simulink model "playground"  (R2024a)
settings: Solver=ode45  StartTime=0.0  StopTime=10.0  FixedStep=0.001  RelTol=1e-3
values from neighbouring files (symbols this model uses):
  a_r = 1.14 * 10^(-7)    (= 1.14e-07)    [start.m]    (also in startEnglPaper.m = 0.033; startReduced.m)
  a_rS = b    (= 0.033)    [startEnglPaper.m]
  A_x = 0.25    [playgrounMat.m]    (also in start.m; startEnglPaper.m; startReduced.m)
  A_y = 0.25    [playgrounMat.m]    (also in start.m; startEnglPaper.m; startReduced.m)
  A_z = 0.25    [playgrounMat.m]    (also in start.m; startEnglPaper.m; startReduced.m)
  b = 1.14 * 10^(-7)    (= 1.14e-07)    [start.m]    (also in startEnglPaper.m = 0.033; startReduced.m)
  g = 9.81    [playgrounMat.m]    (also in start.m; startEnglPaper.m; startReduced.m)
  gamma_d = pi/3    (= 1.0471975512)    [start.m]    (also in startReduced.m)
  I_r = 5.38 * 10 ^ (-5)    (= 5.38e-05)    [start.m]    (also in startEnglPaper.m = 3.38e-05; startReduced.m)
  I_x = 0.0151    [start.m]    (also in startEnglPaper.m = 0.004856; startReduced.m)
  I_y = 0.253    [start.m]    (also in startEnglPaper.m = 0.004856; startReduced.m)
  I_z = 0.0151    [start.m]    (also in startEnglPaper.m = 0.008801; startReduced.m)
  IrS = 5.38 * 10^(-5)    (= 5.38e-05)    [startEnglPaper.m]
  IxS = 0.0151    [startEnglPaper.m]
  IyS = IxS    (= 0.0151)    [startEnglPaper.m]
  IzS = 0.0253    [startEnglPaper.m]
  k = 1.045 * 10^(-11)    (= 1.045e-11)    [start.m]    (also in startEnglPaper.m = 2.98e-06; startReduced.m)
  K_gamma_D1 = K(1)    [playgrounMat.m]
  K_gamma_I1 = K(3)    [playgrounMat.m]
  K_gamma_P1 = K(2)    [playgrounMat.m]
  K_phi_D1 = 0.047    [startEnglPaper.m]
  K_phi_D11 = 0.093    [startEnglPaper.m]
  K_phi_D2 = 9.6    [startEnglPaper.m]
  K_phi_D22 = 19.2    [startEnglPaper.m]
  K_phi_DS = 0.14    [startEnglPaper.m]
  K_phi_I11 = 1.27    [startEnglPaper.m]
  K_phi_I22 = 262.144    [startEnglPaper.m]
  K_phi_P1 = 0.11    [startEnglPaper.m]
  K_phi_P11 = 0.5966    [startEnglPaper.m]
  K_phi_P2 = 23.04    [startEnglPaper.m]
  K_phi_P22 = 122.88    [startEnglPaper.m]
  K_phi_PS = 0.35    [startEnglPaper.m]
  K_psi_D = 40    [start.m]    (also in startEnglPaper.m = 9.6; startReduced.m)
  K_psi_D1 = 0.0844    [startEnglPaper.m]
  K_psi_D2 = 9.6    [startEnglPaper.m]
  K_psi_D22 = 19.2    [startEnglPaper.m]
  K_psi_DS = 0.24    [startEnglPaper.m]
  K_psi_I22 = 262.144    [startEnglPaper.m]
  K_psi_P = 143    [start.m]    (also in startEnglPaper.m = 23.04; startReduced.m)
  K_psi_P1 = 0.202    [startEnglPaper.m]
  K_psi_P2 = 23.04    [startEnglPaper.m]
  K_psi_P22 = 122.88    [startEnglPaper.m]
  K_psi_PS = 0.58    [startEnglPaper.m]
  K_theta_D = 58    [start.m]    (also in startEnglPaper.m = 9.6; startReduced.m)
  K_theta_D1 = 0.047    [startEnglPaper.m]
  K_theta_D2 = 9.6    [startEnglPaper.m]
  K_theta_D22 = 19.2    [startEnglPaper.m]
  K_theta_DS = 0.14    [startEnglPaper.m]
  K_theta_I22 = 262.144    [startEnglPaper.m]
  K_theta_P = 141    [start.m]    (also in startEnglPaper.m = 23.04; startReduced.m)
  K_theta_P1 = 0.11    [startEnglPaper.m]
  K_theta_P2 = 23.04    [startEnglPaper.m]
  K_theta_P22 = 122.88    [startEnglPaper.m]
  K_theta_PS = 0.35    [startEnglPaper.m]
  K_y_D = 13.58    [start.m]    (also in startReduced.m)
  K_y_P = 33.18    [start.m]    (also in startReduced.m)
  K_z_D1 = 4.42    [startEnglPaper.m]
  K_z_D2 = 4.42/m + A_z/m    (= 9.60905349794)    [startEnglPaper.m]
  K_z_DS = 13.58    [startEnglPaper.m]
  K_z_P1 = 11.2    [startEnglPaper.m]
  K_z_P2 = 11.2/m + A_z/m    (= 23.5596707819)    [startEnglPaper.m]
  K_z_PS = 33.18    [startEnglPaper.m]
  kl = 3 * 10^(-6)    (= 3e-06)    [startEnglPaper.m]
  l = 0.225    [start.m]    (also in startEnglPaper.m; startReduced.m)
  m = 1.44    [playgrounMat.m]    (also in start.m; startEnglPaper.m = 0.486; startReduced.m)
  m_s = [1/4 0 -1/(2*l) -1/(4*a_r); 1/4 -1/(2*l) 0 1/(4*a_r); 1/4 0 1/(2*l) -1/(4*a_r); 1/4 1/(2*l) 0 1/(4*a_r)]    [start.m]    (also in startReduced.m)
  mS = 1.44    [startEnglPaper.m]
  phi_d = 0.2    [startEnglPaper.m]
  phi_DesS = 0.2    [startEnglPaper.m]
  phi_init = 0    [startEnglPaper.m]
  phi_iS = 0;   deg2rad(10)    [startEnglPaper.m]
  psi_d = pi/5    (= 0.628318530718)    [start.m]    (also in startEnglPaper.m = 0.15; startReduced.m)
  psi_DesS = 0.15    [startEnglPaper.m]
  psi_init = 0    [startEnglPaper.m]
  psi_iS = 0    [startEnglPaper.m]
  theta_d = pi/4    (= 0.785398163397)    [start.m]    (also in startEnglPaper.m = 0.3; startReduced.m)
  theta_DesS = -0.1 * -3    (= 0.3)    [startEnglPaper.m]
  theta_init = 0    [startEnglPaper.m]
  theta_iS = 0    [startEnglPaper.m]
  x_init = 0    [startEnglPaper.m]
  x_iS = 0    [startEnglPaper.m]
  y_init = 0    [startEnglPaper.m]
  y_iS = 0    [startEnglPaper.m]
  z_d = 0.05 * 0    (= 0)    [startEnglPaper.m]
  z_DesS = 0.1    [startEnglPaper.m]
  z_init = 0    [startEnglPaper.m]
  z_iS = 0.0    (= 0)    [startEnglPaper.m]
undefined symbols (not defined in the file or in its folder): m_s_my
libraries: slpidlib x14
(part 3 of 4)

== system playground/CHANGE_PID/CONTROLLER/PD regulator theta ==
  theta : Inport
  (theta)' : Inport  Port=2
  Altitude controller : slpidlib/PID Controller  Controller=PID  Form=Parallel  TimeDomain=Continuous-time  UseExternalTs=off  SampleTime=-1  IntegratorMethod=Forward Euler  FilterMethod=Forward Euler  ControllerParametersSource=internal  P=K_theta_P1  I=0  UseKiTs=off  D=K_theta_D1  UseExternalDerivativeSource=off  N=100  UseFilter=on  TunerSelectOption=Transfer Function Based (PID Tuner App)  InitialConditionSource=internal  InitialConditionForIntegrator=0  InitialConditionForFilter=0  DifferentiatorICPrevScaledInput=0  ExternalReset=none  TrackingMode=off  Kt=1  LimitOutput=on  SatLimitsSource=internal  UpperSaturationLimit=5  LowerSaturationLimit=-5  LinearizeAsGain=on  AntiWindupMode=none  Kb=1  LimitIntegrator=off  UpperIntegratorSaturationLimit=inf  LowerIntegratorSaturationLimit=-inf  POutMin=[]  POutMax=[]  IOutMin=[]  IOutMax=[]  DOutMin=[]  DOutMax=[]  NOutMin=[]  NOutMax=[]  SumOutMin=[]  SumOutMax=[]  SaturationOutMin=[]  SaturationOutMax=[]  PParamMin=[]  PParamMax=[]  IParamMin=[]  IParamMax=[]  DParamMin=[]  DParamMax=[]  NParamMin=[]  NParamMax=[]  KbParamMin=[]  KbParamMax=[]  KtParamMin=[]  KtParamMax=[]  KbOutMin=[]  KbOutMax=[]  KtOutMin=[]  KtOutMax=[]  IntegratorOutMin=[]  IntegratorOutMax=[]  FilterOutMin=[]  FilterOutMax=[]  SumI1OutMin=[]  SumI1OutMax=[]  SumI2OutMin=[]  SumI2OutMax=[]  SumI3OutMin=[]  SumI3OutMax=[]  SumI4OutMin=[]  SumI4OutMax=[]  SumDOutMin=[]  SumDOutMax=[]  DifferentiatorOutMin=[]  DifferentiatorOutMax=[]  FilterDiffOutCoefMin=[]  FilterDiffOutCoefMax=[]  ReciprocalOutMin=[]  ReciprocalOutMax=[]  SumDenOutMin=[]  SumDenOutMax=[]  SumNumOutMin=[]  SumNumOutMax=[]  DivideOutMin=[]  DivideOutMax=[]  UdiffTsProdOutMin=[]  UdiffTsProdOutMax=[]  NTsProdOutMin=[]  NTsProdOutMax=[]  UintegralTsProdOutMin=[]  UintegralTsProdOutMax=[]  UngainTsProdOutMin=[]  UngainTsProdOutMax=[]  ClampingZeroOutDataTypeStr=Inherit: Inherit via back propagation  ClampingZeroOutMin=[]  ClampingZeroOutMax=[]  FilterDenConstantOutDataTypeStr=Inherit: Inherit via back propagation  FilterDenConstantOutMin=[]  FilterDenConstantOutMax=[]  PCopyOutDataTypeStr=Inherit: Inherit via back propagation  PCopyOutMin=[]  PCopyOutMax=[]  NCopyOutDataTypeStr=Inherit: Inherit via back propagation  NCopyOutMin=[]  NCopyOutMax=[]  IntegratorContinuousStateAttributes=''  IntegratorStateMustResolveToSignalObject=off  IntegratorRTWStateStorageClass=Auto  FilterContinuousStateAttributes=''  FilterStateMustResolveToSignalObject=off  FilterRTWStateStorageClass=Auto  ParallelPVariant=InternalParameters  IdealPVariant=Disabled  IVariant=InternalParameters  DVariant=InternalParameters  IntegratorVariant=Continuous  SatVariant=Enabled  AWVariant=Passthrough  PCopyVariant=Disabled  TRVariant=Disabled  FdbkBlocksVariant=Forward  IdealPFdbkVariant=Disabled  SatFdbkVariant=Disabled  DerivativeFilterVariant=ContFilter  NVariant=InternalParameters  NCopyVariant=Disabled  FilterICVariant=InternalICsFilter  IntegratorICVariant=InternalICs  ExternalResetVariant=Disabled  TRSumVariant=Passthrough  SumFdbkVariant=Disabled  SumVariant=Sum_PID  TsampFilterVariant=InternalTs  TsampNgainVariant=Passthrough  TsampIntegralVariant=Disabled_SignalSpec  ExternalSaturationOutDataTypeStr=Inherit: Same as second input  DerivativeSourceVariant=ErrorSignal
  Constant : Constant  Value=I_y/I_y
  Constant1 : Constant  Value=K_theta_D1
  Constant2 : Constant  Value=theta_d
  Constant4 : Constant  Value=K_theta_P1
  Constant5 : Constant  Value=theta_d
  Current x{,1..3} (4 alike) : Display
  Derivative : Derivative
  Product : Product
  Product1 : Product
  Product2 : Product
  Sum : Sum  Inputs=++|
  Sum1 : Sum  Inputs=|+-
  Sum2 : Sum  Inputs=|+-
  tau_theta : Outport
  wires:
  Product/1 -> Current x3/1, Sum/1
  Constant1/1 -> Product/1
  Product1/1 -> Current x2/1, Sum/2
  Sum1/1 -> Product/2
  Constant4/1 -> Product1/1
  theta/1 -> Sum2/2
  Constant5/1 -> Sum2/1
  Derivative/1 -> Sum1/1
  Constant2/1 -> Derivative/1
  (theta)'/1 -> Sum1/2
  Sum2/1 -> Current x/1, Altitude controller/1, Product1/2
  Product2/1 -> tau_theta/1  "tau_theta"
  Constant/1 -> Product2/2
  Altitude controller/1 -> Current x1/1, Product2/1

== system playground/ST_constants_no_IX/CONTROLLER/PD regulator draft ==
  phi : Inport
  theta : Inport  Port=2
  z : Inport  Port=3
  Altitude controller : slpidlib/PID Controller  Controller=PID  Form=Parallel  TimeDomain=Continuous-time  UseExternalTs=off  SampleTime=-1  IntegratorMethod=Forward Euler  FilterMethod=Forward Euler  ControllerParametersSource=internal  P=K_z_PS  I=0  UseKiTs=off  D=K_z_DS  UseExternalDerivativeSource=off  N=100  UseFilter=on  TunerSelectOption=Transfer Function Based (PID Tuner App)  InitialConditionSource=internal  InitialConditionForIntegrator=0  InitialConditionForFilter=0  DifferentiatorICPrevScaledInput=0  ExternalReset=none  TrackingMode=off  Kt=1  LimitOutput=on  SatLimitsSource=internal  UpperSaturationLimit=5  LowerSaturationLimit=-5  LinearizeAsGain=on  AntiWindupMode=none  Kb=1  LimitIntegrator=off  UpperIntegratorSaturationLimit=inf  LowerIntegratorSaturationLimit=-inf  POutMin=[]  POutMax=[]  IOutMin=[]  IOutMax=[]  DOutMin=[]  DOutMax=[]  NOutMin=[]  NOutMax=[]  SumOutMin=[]  SumOutMax=[]  SaturationOutMin=[]  SaturationOutMax=[]  PParamMin=[]  PParamMax=[]  IParamMin=[]  IParamMax=[]  DParamMin=[]  DParamMax=[]  NParamMin=[]  NParamMax=[]  KbParamMin=[]  KbParamMax=[]  KtParamMin=[]  KtParamMax=[]  KbOutMin=[]  KbOutMax=[]  KtOutMin=[]  KtOutMax=[]  IntegratorOutMin=[]  IntegratorOutMax=[]  FilterOutMin=[]  FilterOutMax=[]  SumI1OutMin=[]  SumI1OutMax=[]  SumI2OutMin=[]  SumI2OutMax=[]  SumI3OutMin=[]  SumI3OutMax=[]  SumI4OutMin=[]  SumI4OutMax=[]  SumDOutMin=[]  SumDOutMax=[]  DifferentiatorOutMin=[]  DifferentiatorOutMax=[]  FilterDiffOutCoefMin=[]  FilterDiffOutCoefMax=[]  ReciprocalOutMin=[]  ReciprocalOutMax=[]  SumDenOutMin=[]  SumDenOutMax=[]  SumNumOutMin=[]  SumNumOutMax=[]  DivideOutMin=[]  DivideOutMax=[]  UdiffTsProdOutMin=[]  UdiffTsProdOutMax=[]  NTsProdOutMin=[]  NTsProdOutMax=[]  UintegralTsProdOutMin=[]  UintegralTsProdOutMax=[]  UngainTsProdOutMin=[]  UngainTsProdOutMax=[]  ClampingZeroOutDataTypeStr=Inherit: Inherit via back propagation  ClampingZeroOutMin=[]  ClampingZeroOutMax=[]  FilterDenConstantOutDataTypeStr=Inherit: Inherit via back propagation  FilterDenConstantOutMin=[]  FilterDenConstantOutMax=[]  PCopyOutDataTypeStr=Inherit: Inherit via back propagation  PCopyOutMin=[]  PCopyOutMax=[]  NCopyOutDataTypeStr=Inherit: Inherit via back propagation  NCopyOutMin=[]  NCopyOutMax=[]  IntegratorContinuousStateAttributes=''  IntegratorStateMustResolveToSignalObject=off  IntegratorRTWStateStorageClass=Auto  FilterContinuousStateAttributes=''  FilterStateMustResolveToSignalObject=off  FilterRTWStateStorageClass=Auto  ParallelPVariant=InternalParameters  IdealPVariant=Disabled  IVariant=InternalParameters  DVariant=InternalParameters  IntegratorVariant=Continuous  SatVariant=Enabled  AWVariant=Passthrough  PCopyVariant=Disabled  TRVariant=Disabled  FdbkBlocksVariant=Forward  IdealPFdbkVariant=Disabled  SatFdbkVariant=Disabled  DerivativeFilterVariant=ContFilter  NVariant=InternalParameters  NCopyVariant=Disabled  FilterICVariant=InternalICsFilter  IntegratorICVariant=InternalICs  ExternalResetVariant=Disabled  TRSumVariant=Passthrough  SumFdbkVariant=Disabled  SumVariant=Sum_PID  TsampFilterVariant=InternalTs  TsampNgainVariant=Passthrough  TsampIntegralVariant=Disabled_SignalSpec  ExternalSaturationOutDataTypeStr=Inherit: Same as second input  DerivativeSourceVariant=ErrorSignal
  Constant : Constant  Value=g
  Constant7 : Constant  Value=mS
  Derivative1 : Derivative
  Derivative2 : Derivative
  Display1 : Display
  Display2 : Display
  Display3 : Display
  Gain : Gain  Gain=K_z_D2
  Gain1 : Gain  Gain=K_z_P2
  Product4 : Product
  Sum : Sum  Inputs=+++
  Sum1 : Sum  Inputs=|+-
  Sum2 : Sum  Inputs=|-+
  m/cos(y)*(cos(theta)) : MATLAB Function  TreatAsAtomicUnit=on
  target2 : Constant  Value=z_d
  target3 : Constant  Value=z_DesS
  T : Outport
  wires:
  Altitude controller/1 -> Sum/3
  Gain1/1 -> Display2/1
  target3/1 -> Sum2/2
  Gain/1 -> Display1/1
  target2/1 -> Derivative2/1
  m/cos(y)*(cos(theta))/1(c) -> Product4/2
  Constant7/1 -> m/cos(y)*(cos(theta))/1(m)
  Sum1/1 -> Gain/1
  z/1 -> Display3/1, Sum2/1, Derivative1/1  "z"
  Derivative1/1 -> Sum1/2
  Constant/1 -> Sum/2
  Derivative2/1 -> Sum1/1
  Sum2/1 -> Gain1/1, Altitude controller/1
  theta/1 -> m/cos(y)*(cos(theta))/3(theta)  "theta"
  phi/1 -> m/cos(y)*(cos(theta))/2(phi)  "gamma"
  Sum/1 -> Product4/1
  Product4/1 -> T/1  "T"

== system playground/ST_constants_no_IX/CONTROLLER/PD regulator gamma1 ==
  phi : Inport
  (phi)' : Inport  Port=2
  Constant : Constant  Value=IxS/IxS
  Constant2 : Constant  Value=phi_DesS
  Constant5 : Constant  Value=phi_DesS
  Current x : Display
  Derivative : Derivative
  Gain : Gain  Gain=K_phi_DS
  Gain1 : Gain  Gain=K_phi_PS
  Product2 : Product
  Sum : Sum  Inputs=++|
  Sum1 : Sum  Inputs=|+-
  Sum2 : Sum  Inputs=|+-
  tau_phi : Outport
  wires:
  Gain1/1 -> Sum/2
  Sum2/1 -> Gain1/1
  Gain/1 -> Sum/1
  Product2/1 -> tau_phi/1  "tau_gamma"
  Sum1/1 -> Gain/1
  phi/1 -> Sum2/2
  Constant5/1 -> Sum2/1
  Derivative/1 -> Sum1/1
  Constant2/1 -> Derivative/1
  (phi)'/1 -> Sum1/2
  Constant/1 -> Product2/2
  Sum/1 -> Current x/1, Product2/1

== system playground/ST_constants_no_IX/CONTROLLER/PD regulator psi ==
  psi : Inport
  (psi)' : Inport  Port=2
  Constant : Constant  Value=IzS/IzS
  Constant1 : Constant  Value=K_psi_DS
  Constant2 : Constant  Value=psi_DesS
  Constant4 : Constant  Value=K_psi_PS
  Constant5 : Constant  Value=psi_DesS
  Derivative : Derivative
  Product : Product
  Product1 : Product
  Product2 : Product
  Sum : Sum  Inputs=++|
  Sum1 : Sum  Inputs=|+-
  Sum2 : Sum  Inputs=|+-
  tau_psi : Outport
  wires:
  Product/1 -> Sum/1
  Constant1/1 -> Product/1
  Product1/1 -> Sum/2
  Sum1/1 -> Product/2
  Constant4/1 -> Product1/1
  psi/1 -> Sum2/2
  Constant5/1 -> Sum2/1
  Derivative/1 -> Sum1/1
  Constant2/1 -> Derivative/1
  (psi)'/1 -> Sum1/2
  Sum2/1 -> Product1/2
  Product2/1 -> tau_psi/1  "tau_psi"
  Constant/1 -> Product2/2
  Sum/1 -> Product2/1

== system playground/ST_constants_no_IX/CONTROLLER/PD regulator theta ==
  theta : Inport
  (theta)' : Inport  Port=2
  Constant : Constant  Value=IyS/IyS
  Constant1 : Constant  Value=K_theta_DS
  Constant2 : Constant  Value=theta_DesS
  Constant4 : Constant  Value=K_theta_PS
  Constant5 : Constant  Value=theta_DesS
  Derivative : Derivative
  Product : Product
  Product1 : Product
  Product2 : Product
  Sum : Sum  Inputs=++|
  Sum1 : Sum  Inputs=|+-
  Sum2 : Sum  Inputs=|+-
  tau_theta : Outport
  wires:
  Product/1 -> Sum/1
  Constant1/1 -> Product/1
  Product1/1 -> Sum/2
  Sum1/1 -> Product/2
  Constant4/1 -> Product1/1
  theta/1 -> Sum2/2
  Constant5/1 -> Sum2/1
  Derivative/1 -> Sum1/1
  Constant2/1 -> Derivative/1
  (theta)'/1 -> Sum1/2
  Sum2/1 -> Product1/2
  Product2/1 -> tau_theta/1  "tau_theta"
  Constant/1 -> Product2/2
  Sum/1 -> Product2/1

== system playground/ST_constants_useIX/CONTROLLER/PD regulator draft ==
  phi : Inport
  theta : Inport  Port=2
  z : Inport  Port=3
  Altitude controller : slpidlib/PID Controller  Controller=PID  Form=Parallel  TimeDomain=Continuous-time  UseExternalTs=off  SampleTime=-1  IntegratorMethod=Forward Euler  FilterMethod=Forward Euler  ControllerParametersSource=internal  P=K_z_PS  I=0  UseKiTs=off  D=K_z_DS  UseExternalDerivativeSource=off  N=100  UseFilter=on  TunerSelectOption=Transfer Function Based (PID Tuner App)  InitialConditionSource=internal  InitialConditionForIntegrator=0  InitialConditionForFilter=0  DifferentiatorICPrevScaledInput=0  ExternalReset=none  TrackingMode=off  Kt=1  LimitOutput=on  SatLimitsSource=internal  UpperSaturationLimit=5  LowerSaturationLimit=-5  LinearizeAsGain=on  AntiWindupMode=none  Kb=1  LimitIntegrator=off  UpperIntegratorSaturationLimit=inf  LowerIntegratorSaturationLimit=-inf  POutMin=[]  POutMax=[]  IOutMin=[]  IOutMax=[]  DOutMin=[]  DOutMax=[]  NOutMin=[]  NOutMax=[]  SumOutMin=[]  SumOutMax=[]  SaturationOutMin=[]  SaturationOutMax=[]  PParamMin=[]  PParamMax=[]  IParamMin=[]  IParamMax=[]  DParamMin=[]  DParamMax=[]  NParamMin=[]  NParamMax=[]  KbParamMin=[]  KbParamMax=[]  KtParamMin=[]  KtParamMax=[]  KbOutMin=[]  KbOutMax=[]  KtOutMin=[]  KtOutMax=[]  IntegratorOutMin=[]  IntegratorOutMax=[]  FilterOutMin=[]  FilterOutMax=[]  SumI1OutMin=[]  SumI1OutMax=[]  SumI2OutMin=[]  SumI2OutMax=[]  SumI3OutMin=[]  SumI3OutMax=[]  SumI4OutMin=[]  SumI4OutMax=[]  SumDOutMin=[]  SumDOutMax=[]  DifferentiatorOutMin=[]  DifferentiatorOutMax=[]  FilterDiffOutCoefMin=[]  FilterDiffOutCoefMax=[]  ReciprocalOutMin=[]  ReciprocalOutMax=[]  SumDenOutMin=[]  SumDenOutMax=[]  SumNumOutMin=[]  SumNumOutMax=[]  DivideOutMin=[]  DivideOutMax=[]  UdiffTsProdOutMin=[]  UdiffTsProdOutMax=[]  NTsProdOutMin=[]  NTsProdOutMax=[]  UintegralTsProdOutMin=[]  UintegralTsProdOutMax=[]  UngainTsProdOutMin=[]  UngainTsProdOutMax=[]  ClampingZeroOutDataTypeStr=Inherit: Inherit via back propagation  ClampingZeroOutMin=[]  ClampingZeroOutMax=[]  FilterDenConstantOutDataTypeStr=Inherit: Inherit via back propagation  FilterDenConstantOutMin=[]  FilterDenConstantOutMax=[]  PCopyOutDataTypeStr=Inherit: Inherit via back propagation  PCopyOutMin=[]  PCopyOutMax=[]  NCopyOutDataTypeStr=Inherit: Inherit via back propagation  NCopyOutMin=[]  NCopyOutMax=[]  IntegratorContinuousStateAttributes=''  IntegratorStateMustResolveToSignalObject=off  IntegratorRTWStateStorageClass=Auto  FilterContinuousStateAttributes=''  FilterStateMustResolveToSignalObject=off  FilterRTWStateStorageClass=Auto  ParallelPVariant=InternalParameters  IdealPVariant=Disabled  IVariant=InternalParameters  DVariant=InternalParameters  IntegratorVariant=Continuous  SatVariant=Enabled  AWVariant=Passthrough  PCopyVariant=Disabled  TRVariant=Disabled  FdbkBlocksVariant=Forward  IdealPFdbkVariant=Disabled  SatFdbkVariant=Disabled  DerivativeFilterVariant=ContFilter  NVariant=InternalParameters  NCopyVariant=Disabled  FilterICVariant=InternalICsFilter  IntegratorICVariant=InternalICs  ExternalResetVariant=Disabled  TRSumVariant=Passthrough  SumFdbkVariant=Disabled  SumVariant=Sum_PID  TsampFilterVariant=InternalTs  TsampNgainVariant=Passthrough  TsampIntegralVariant=Disabled_SignalSpec  ExternalSaturationOutDataTypeStr=Inherit: Same as second input  DerivativeSourceVariant=ErrorSignal
  Constant : Constant  Value=g
  Constant7 : Constant  Value=mS
  Derivative1 : Derivative
  Derivative2 : Derivative
  Display1 : Display
  Display2 : Display
  Display3 : Display
  Gain : Gain  Gain=K_z_D2
  Gain1 : Gain  Gain=K_z_P2
  Product4 : Product
  Sum : Sum  Inputs=+++
  Sum1 : Sum  Inputs=|+-
  Sum2 : Sum  Inputs=|-+
  m/cos(y)*(cos(theta)) : MATLAB Function  TreatAsAtomicUnit=on
  target2 : Constant  Value=z_d
  target3 : Constant  Value=z_DesS
  T : Outport
  wires:
  Product4/1 -> T/1  "T"
  Sum/1 -> Product4/1
  phi/1 -> m/cos(y)*(cos(theta))/2(phi)  "gamma"
  theta/1 -> m/cos(y)*(cos(theta))/3(theta)  "theta"
  Sum2/1 -> Altitude controller/1, Gain1/1
  Derivative2/1 -> Sum1/1
  Constant/1 -> Sum/2
  Derivative1/1 -> Sum1/2
  z/1 -> Derivative1/1, Sum2/1, Display3/1  "z"
  Sum1/1 -> Gain/1
  Constant7/1 -> m/cos(y)*(cos(theta))/1(m)
  m/cos(y)*(cos(theta))/1(c) -> Product4/2
  target2/1 -> Derivative2/1
  Gain/1 -> Display1/1
  target3/1 -> Sum2/2
  Gain1/1 -> Display2/1
  Altitude controller/1 -> Sum/3

== system playground/ST_constants_useIX/CONTROLLER/PD regulator gamma1 ==
  phi : Inport
  (phi)' : Inport  Port=2
  Altitude controller1 : slpidlib/PID Controller  Controller=PID  Form=Parallel  TimeDomain=Continuous-time  UseExternalTs=off  SampleTime=-1  IntegratorMethod=Forward Euler  FilterMethod=Forward Euler  ControllerParametersSource=internal  P=122.88  I=262.14  UseKiTs=off  D=19.2  UseExternalDerivativeSource=off  N=100  UseFilter=on  TunerSelectOption=Transfer Function Based (PID Tuner App)  InitialConditionSource=internal  InitialConditionForIntegrator=0  InitialConditionForFilter=0  DifferentiatorICPrevScaledInput=0  ExternalReset=none  TrackingMode=off  Kt=1  LimitOutput=on  SatLimitsSource=internal  UpperSaturationLimit=15  LowerSaturationLimit=-15  LinearizeAsGain=on  AntiWindupMode=none  Kb=1  LimitIntegrator=off  UpperIntegratorSaturationLimit=inf  LowerIntegratorSaturationLimit=-inf  POutMin=[]  POutMax=[]  IOutMin=[]  IOutMax=[]  DOutMin=[]  DOutMax=[]  NOutMin=[]  NOutMax=[]  SumOutMin=[]  SumOutMax=[]  SaturationOutMin=[]  SaturationOutMax=[]  PParamMin=[]  PParamMax=[]  IParamMin=[]  IParamMax=[]  DParamMin=[]  DParamMax=[]  NParamMin=[]  NParamMax=[]  KbParamMin=[]  KbParamMax=[]  KtParamMin=[]  KtParamMax=[]  KbOutMin=[]  KbOutMax=[]  KtOutMin=[]  KtOutMax=[]  IntegratorOutMin=[]  IntegratorOutMax=[]  FilterOutMin=[]  FilterOutMax=[]  SumI1OutMin=[]  SumI1OutMax=[]  SumI2OutMin=[]  SumI2OutMax=[]  SumI3OutMin=[]  SumI3OutMax=[]  SumI4OutMin=[]  SumI4OutMax=[]  SumDOutMin=[]  SumDOutMax=[]  DifferentiatorOutMin=[]  DifferentiatorOutMax=[]  FilterDiffOutCoefMin=[]  FilterDiffOutCoefMax=[]  ReciprocalOutMin=[]  ReciprocalOutMax=[]  SumDenOutMin=[]  SumDenOutMax=[]  SumNumOutMin=[]  SumNumOutMax=[]  DivideOutMin=[]  DivideOutMax=[]  UdiffTsProdOutMin=[]  UdiffTsProdOutMax=[]  NTsProdOutMin=[]  NTsProdOutMax=[]  UintegralTsProdOutMin=[]  UintegralTsProdOutMax=[]  UngainTsProdOutMin=[]  UngainTsProdOutMax=[]  ClampingZeroOutDataTypeStr=Inherit: Inherit via back propagation  ClampingZeroOutMin=[]  ClampingZeroOutMax=[]  FilterDenConstantOutDataTypeStr=Inherit: Inherit via back propagation  FilterDenConstantOutMin=[]  FilterDenConstantOutMax=[]  PCopyOutDataTypeStr=Inherit: Inherit via back propagation  PCopyOutMin=[]  PCopyOutMax=[]  NCopyOutDataTypeStr=Inherit: Inherit via back propagation  NCopyOutMin=[]  NCopyOutMax=[]  IntegratorContinuousStateAttributes=''  IntegratorStateMustResolveToSignalObject=off  IntegratorRTWStateStorageClass=Auto  FilterContinuousStateAttributes=''  FilterStateMustResolveToSignalObject=off  FilterRTWStateStorageClass=Auto  ParallelPVariant=InternalParameters  IdealPVariant=Disabled  IVariant=InternalParameters  DVariant=InternalParameters  IntegratorVariant=Continuous  SatVariant=Enabled  AWVariant=Passthrough  PCopyVariant=Disabled  TRVariant=Disabled  FdbkBlocksVariant=Forward  IdealPFdbkVariant=Disabled  SatFdbkVariant=Disabled  DerivativeFilterVariant=ContFilter  NVariant=InternalParameters  NCopyVariant=Disabled  FilterICVariant=InternalICsFilter  IntegratorICVariant=InternalICs  ExternalResetVariant=Disabled  TRSumVariant=Passthrough  SumFdbkVariant=Disabled  SumVariant=Sum_PID  TsampFilterVariant=InternalTs  TsampNgainVariant=Passthrough  TsampIntegralVariant=Disabled_SignalSpec  ExternalSaturationOutDataTypeStr=Inherit: Same as second input  DerivativeSourceVariant=ErrorSignal
  Constant : Constant  Value=IxS
  Constant2 : Constant  Value=phi_DesS
  Constant5 : Constant  Value=phi_DesS
  Current x : Display
  Derivative : Derivative
  Gain : Gain  Gain=9.6
  Gain1 : Gain  Gain=23.04
  Manual Switch1 : ManualSwitch
  Manual Switch2 : ManualSwitch  CurrentSetting=0
  Manual Switch3 : ManualSwitch  CurrentSetting=0
  PID hand : Subsystem
  Product2 : Product
  Sum : Sum  Inputs=++|
  Sum1 : Sum  Inputs=|+-
  Sum2 : Sum  Inputs=|+-
  Sum3 : Sum  Inputs=|+-
  Фильтр ПИД3 : TransferFcn  Numerator=[262.14]  Denominator=[19.2 122.88 262.14]
  tau_phi : Outport
  wires:
  Sum/1 -> Manual Switch2/1, Current x/1
  Constant/1 -> Product2/2
  (phi)'/1 -> Sum1/2
  Constant2/1 -> Derivative/1
  Derivative/1 -> Sum1/1
  Constant5/1 -> Фильтр ПИД3/1, Sum2/1
  phi/1 -> Sum2/2, Sum3/2
  Sum1/1 -> Gain/1
  Product2/1 -> tau_phi/1  "tau_gamma"
  Gain/1 -> Sum/1
  Sum2/1 -> Manual Switch1/1, Gain1/1
  Gain1/1 -> Sum/2
  Manual Switch1/1 -> PID hand/1(err), Altitude controller1/1
  Manual Switch2/1 -> Product2/1
  Altitude controller1/1 -> Manual Switch3/1
  Фильтр ПИД3/1 -> Sum3/1
  Sum3/1 -> Manual Switch1/2
  PID hand/1(res) -> Manual Switch3/2
  Manual Switch3/1 -> Manual Switch2/2

== system playground/ST_constants_useIX/CONTROLLER/PD regulator psi ==
  psi : Inport
  (psi)' : Inport  Port=2
  Altitude controller1 : slpidlib/PID Controller  Controller=PID  Form=Parallel  TimeDomain=Continuous-time  UseExternalTs=off  SampleTime=-1  IntegratorMethod=Forward Euler  FilterMethod=Forward Euler  ControllerParametersSource=internal  P=122.88  I=262.14  UseKiTs=off  D=19.2  UseExternalDerivativeSource=off  N=100  UseFilter=on  TunerSelectOption=Transfer Function Based (PID Tuner App)  InitialConditionSource=internal  InitialConditionForIntegrator=0  InitialConditionForFilter=0  DifferentiatorICPrevScaledInput=0  ExternalReset=none  TrackingMode=off  Kt=1  LimitOutput=on  SatLimitsSource=internal  UpperSaturationLimit=5  LowerSaturationLimit=-5  LinearizeAsGain=on  AntiWindupMode=none  Kb=1  LimitIntegrator=off  UpperIntegratorSaturationLimit=inf  LowerIntegratorSaturationLimit=-inf  POutMin=[]  POutMax=[]  IOutMin=[]  IOutMax=[]  DOutMin=[]  DOutMax=[]  NOutMin=[]  NOutMax=[]  SumOutMin=[]  SumOutMax=[]  SaturationOutMin=[]  SaturationOutMax=[]  PParamMin=[]  PParamMax=[]  IParamMin=[]  IParamMax=[]  DParamMin=[]  DParamMax=[]  NParamMin=[]  NParamMax=[]  KbParamMin=[]  KbParamMax=[]  KtParamMin=[]  KtParamMax=[]  KbOutMin=[]  KbOutMax=[]  KtOutMin=[]  KtOutMax=[]  IntegratorOutMin=[]  IntegratorOutMax=[]  FilterOutMin=[]  FilterOutMax=[]  SumI1OutMin=[]  SumI1OutMax=[]  SumI2OutMin=[]  SumI2OutMax=[]  SumI3OutMin=[]  SumI3OutMax=[]  SumI4OutMin=[]  SumI4OutMax=[]  SumDOutMin=[]  SumDOutMax=[]  DifferentiatorOutMin=[]  DifferentiatorOutMax=[]  FilterDiffOutCoefMin=[]  FilterDiffOutCoefMax=[]  ReciprocalOutMin=[]  ReciprocalOutMax=[]  SumDenOutMin=[]  SumDenOutMax=[]  SumNumOutMin=[]  SumNumOutMax=[]  DivideOutMin=[]  DivideOutMax=[]  UdiffTsProdOutMin=[]  UdiffTsProdOutMax=[]  NTsProdOutMin=[]  NTsProdOutMax=[]  UintegralTsProdOutMin=[]  UintegralTsProdOutMax=[]  UngainTsProdOutMin=[]  UngainTsProdOutMax=[]  ClampingZeroOutDataTypeStr=Inherit: Inherit via back propagation  ClampingZeroOutMin=[]  ClampingZeroOutMax=[]  FilterDenConstantOutDataTypeStr=Inherit: Inherit via back propagation  FilterDenConstantOutMin=[]  FilterDenConstantOutMax=[]  PCopyOutDataTypeStr=Inherit: Inherit via back propagation  PCopyOutMin=[]  PCopyOutMax=[]  NCopyOutDataTypeStr=Inherit: Inherit via back propagation  NCopyOutMin=[]  NCopyOutMax=[]  IntegratorContinuousStateAttributes=''  IntegratorStateMustResolveToSignalObject=off  IntegratorRTWStateStorageClass=Auto  FilterContinuousStateAttributes=''  FilterStateMustResolveToSignalObject=off  FilterRTWStateStorageClass=Auto  ParallelPVariant=InternalParameters  IdealPVariant=Disabled  IVariant=InternalParameters  DVariant=InternalParameters  IntegratorVariant=Continuous  SatVariant=Enabled  AWVariant=Passthrough  PCopyVariant=Disabled  TRVariant=Disabled  FdbkBlocksVariant=Forward  IdealPFdbkVariant=Disabled  SatFdbkVariant=Disabled  DerivativeFilterVariant=ContFilter  NVariant=InternalParameters  NCopyVariant=Disabled  FilterICVariant=InternalICsFilter  IntegratorICVariant=InternalICs  ExternalResetVariant=Disabled  TRSumVariant=Passthrough  SumFdbkVariant=Disabled  SumVariant=Sum_PID  TsampFilterVariant=InternalTs  TsampNgainVariant=Passthrough  TsampIntegralVariant=Disabled_SignalSpec  ExternalSaturationOutDataTypeStr=Inherit: Same as second input  DerivativeSourceVariant=ErrorSignal
  Constant : Constant  Value=IzS
  Constant1 : Constant  Value=K_psi_DS
  Constant2 : Constant  Value=psi_DesS
  Constant4 : Constant  Value=K_psi_PS
  Constant5 : Constant  Value=psi_DesS
  Derivative : Derivative
  Manual Switch1 : ManualSwitch  CurrentSetting=0
  Manual Switch2 : ManualSwitch
  Product : Product
  Product1 : Product
  Product2 : Product
  Sum : Sum  Inputs=++|
  Sum1 : Sum  Inputs=|+-
  Sum2 : Sum  Inputs=|+-
  Sum3 : Sum  Inputs=|+-
  Фильтр ПИД1 : TransferFcn  Numerator=[262.14]  Denominator=[19.2 122.88 262.14]
  tau_psi : Outport
  wires:
  Sum/1 -> Manual Switch1/1
  Constant/1 -> Product2/2
  Product2/1 -> tau_psi/1  "tau_psi"
  (psi)'/1 -> Sum1/2
  Constant2/1 -> Derivative/1
  Derivative/1 -> Sum1/1
  Constant5/1 -> Фильтр ПИД1/1, Sum2/1
  Constant4/1 -> Product1/1
  Sum1/1 -> Product/2
  Product1/1 -> Sum/2
  Constant1/1 -> Product/1
  Product/1 -> Sum/1
  Sum3/1 -> Manual Switch2/2
  Altitude controller1/1 -> Manual Switch1/2
  Manual Switch2/1 -> Altitude controller1/1
  Фильтр ПИД1/1 -> Sum3/1
  psi/1 -> Sum2/2, Sum3/2
  Sum2/1 -> Manual Switch2/1, Product1/2
  Manual Switch1/1 -> Product2/1

== system playground/ST_constants_useIX/CONTROLLER/PD regulator theta ==
  theta : Inport
  (theta)' : Inport  Port=2
  Altitude controller1 : slpidlib/PID Controller  Controller=PID  Form=Parallel  TimeDomain=Continuous-time  UseExternalTs=off  SampleTime=-1  IntegratorMethod=Forward Euler  FilterMethod=Forward Euler  ControllerParametersSource=internal  P=122.88  I=262.14  UseKiTs=off  D=19.2  UseExternalDerivativeSource=off  N=100  UseFilter=on  TunerSelectOption=Transfer Function Based (PID Tuner App)  InitialConditionSource=internal  InitialConditionForIntegrator=0  InitialConditionForFilter=0  DifferentiatorICPrevScaledInput=0  ExternalReset=none  TrackingMode=off  Kt=1  LimitOutput=on  SatLimitsSource=internal  UpperSaturationLimit=15  LowerSaturationLimit=-10  LinearizeAsGain=on  AntiWindupMode=none  Kb=1  LimitIntegrator=off  UpperIntegratorSaturationLimit=inf  LowerIntegratorSaturationLimit=-inf  POutMin=[]  POutMax=[]  IOutMin=[]  IOutMax=[]  DOutMin=[]  DOutMax=[]  NOutMin=[]  NOutMax=[]  SumOutMin=[]  SumOutMax=[]  SaturationOutMin=[]  SaturationOutMax=[]  PParamMin=[]  PParamMax=[]  IParamMin=[]  IParamMax=[]  DParamMin=[]  DParamMax=[]  NParamMin=[]  NParamMax=[]  KbParamMin=[]  KbParamMax=[]  KtParamMin=[]  KtParamMax=[]  KbOutMin=[]  KbOutMax=[]  KtOutMin=[]  KtOutMax=[]  IntegratorOutMin=[]  IntegratorOutMax=[]  FilterOutMin=[]  FilterOutMax=[]  SumI1OutMin=[]  SumI1OutMax=[]  SumI2OutMin=[]  SumI2OutMax=[]  SumI3OutMin=[]  SumI3OutMax=[]  SumI4OutMin=[]  SumI4OutMax=[]  SumDOutMin=[]  SumDOutMax=[]  DifferentiatorOutMin=[]  DifferentiatorOutMax=[]  FilterDiffOutCoefMin=[]  FilterDiffOutCoefMax=[]  ReciprocalOutMin=[]  ReciprocalOutMax=[]  SumDenOutMin=[]  SumDenOutMax=[]  SumNumOutMin=[]  SumNumOutMax=[]  DivideOutMin=[]  DivideOutMax=[]  UdiffTsProdOutMin=[]  UdiffTsProdOutMax=[]  NTsProdOutMin=[]  NTsProdOutMax=[]  UintegralTsProdOutMin=[]  UintegralTsProdOutMax=[]  UngainTsProdOutMin=[]  UngainTsProdOutMax=[]  ClampingZeroOutDataTypeStr=Inherit: Inherit via back propagation  ClampingZeroOutMin=[]  ClampingZeroOutMax=[]  FilterDenConstantOutDataTypeStr=Inherit: Inherit via back propagation  FilterDenConstantOutMin=[]  FilterDenConstantOutMax=[]  PCopyOutDataTypeStr=Inherit: Inherit via back propagation  PCopyOutMin=[]  PCopyOutMax=[]  NCopyOutDataTypeStr=Inherit: Inherit via back propagation  NCopyOutMin=[]  NCopyOutMax=[]  IntegratorContinuousStateAttributes=''  IntegratorStateMustResolveToSignalObject=off  IntegratorRTWStateStorageClass=Auto  FilterContinuousStateAttributes=''  FilterStateMustResolveToSignalObject=off  FilterRTWStateStorageClass=Auto  ParallelPVariant=InternalParameters  IdealPVariant=Disabled  IVariant=InternalParameters  DVariant=InternalParameters  IntegratorVariant=Continuous  SatVariant=Enabled  AWVariant=Passthrough  PCopyVariant=Disabled  TRVariant=Disabled  FdbkBlocksVariant=Forward  IdealPFdbkVariant=Disabled  SatFdbkVariant=Disabled  DerivativeFilterVariant=ContFilter  NVariant=InternalParameters  NCopyVariant=Disabled  FilterICVariant=InternalICsFilter  IntegratorICVariant=InternalICs  ExternalResetVariant=Disabled  TRSumVariant=Passthrough  SumFdbkVariant=Disabled  SumVariant=Sum_PID  TsampFilterVariant=InternalTs  TsampNgainVariant=Passthrough  TsampIntegralVariant=Disabled_SignalSpec  ExternalSaturationOutDataTypeStr=Inherit: Same as second input  DerivativeSourceVariant=ErrorSignal
  Constant : Constant  Value=IyS
  Constant1 : Constant  Value=K_theta_DS
  Constant2 : Constant  Value=theta_DesS
  Constant4 : Constant  Value=K_theta_PS
  Constant5 : Constant  Value=theta_DesS
  Derivative : Derivative
  Manual Switch2 : ManualSwitch
  Manual Switch3 : ManualSwitch  CurrentSetting=0
  Product : Product
  Product1 : Product
  Product2 : Product
  Sum : Sum  Inputs=++|
  Sum1 : Sum  Inputs=|+-
  Sum2 : Sum  Inputs=|+-
  Sum3 : Sum  Inputs=|+-
  Фильтр ПИД1 : TransferFcn  Numerator=[262.14]  Denominator=[19.2 122.88 262.14]
  tau_theta : Outport
  wires:
  Constant/1 -> Product2/2
  Product2/1 -> tau_theta/1  "tau_theta"
  Sum2/1 -> Manual Switch2/1, Product1/2
  (theta)'/1 -> Sum1/2
  Constant2/1 -> Derivative/1
  Derivative/1 -> Sum1/1
  Constant5/1 -> Sum2/1, Фильтр ПИД1/1
  Constant4/1 -> Product1/1
  Sum1/1 -> Product/2
  Product1/1 -> Sum/2
  Constant1/1 -> Product/1
  Product/1 -> Sum/1
  Фильтр ПИД1/1 -> Sum3/1
  theta/1 -> Sum2/2, Sum3/2
  Sum3/1 -> Manual Switch2/2
  Sum/1 -> Manual Switch3/1
  Manual Switch3/1 -> Product2/1
  Altitude controller1/1 -> Manual Switch3/2
  Manual Switch2/1 -> Altitude controller1/1

== system playground/quad_PID_Simpl2/CONTROLLER/PD regulator draft ==
  phi : Inport
  theta : Inport  Port=2
  z : Inport  Port=3
  Altitude controller : slpidlib/PID Controller  Controller=PID  Form=Parallel  TimeDomain=Continuous-time  UseExternalTs=off  SampleTime=-1  IntegratorMethod=Forward Euler  FilterMethod=Forward Euler  ControllerParametersSource=internal  P=K_z_P2  I=0  UseKiTs=off  D=K_z_D2  UseExternalDerivativeSource=off  N=100  UseFilter=on  TunerSelectOption=Transfer Function Based (PID Tuner App)  InitialConditionSource=internal  InitialConditionForIntegrator=0  InitialConditionForFilter=0  DifferentiatorICPrevScaledInput=0  ExternalReset=none  TrackingMode=off  Kt=1  LimitOutput=on  SatLimitsSource=internal  UpperSaturationLimit=5  LowerSaturationLimit=-5  LinearizeAsGain=on  AntiWindupMode=none  Kb=1  LimitIntegrator=off  UpperIntegratorSaturationLimit=inf  LowerIntegratorSaturationLimit=-inf  POutMin=[]  POutMax=[]  IOutMin=[]  IOutMax=[]  DOutMin=[]  DOutMax=[]  NOutMin=[]  NOutMax=[]  SumOutMin=[]  SumOutMax=[]  SaturationOutMin=[]  SaturationOutMax=[]  PParamMin=[]  PParamMax=[]  IParamMin=[]  IParamMax=[]  DParamMin=[]  DParamMax=[]  NParamMin=[]  NParamMax=[]  KbParamMin=[]  KbParamMax=[]  KtParamMin=[]  KtParamMax=[]  KbOutMin=[]  KbOutMax=[]  KtOutMin=[]  KtOutMax=[]  IntegratorOutMin=[]  IntegratorOutMax=[]  FilterOutMin=[]  FilterOutMax=[]  SumI1OutMin=[]  SumI1OutMax=[]  SumI2OutMin=[]  SumI2OutMax=[]  SumI3OutMin=[]  SumI3OutMax=[]  SumI4OutMin=[]  SumI4OutMax=[]  SumDOutMin=[]  SumDOutMax=[]  DifferentiatorOutMin=[]  DifferentiatorOutMax=[]  FilterDiffOutCoefMin=[]  FilterDiffOutCoefMax=[]  ReciprocalOutMin=[]  ReciprocalOutMax=[]  SumDenOutMin=[]  SumDenOutMax=[]  SumNumOutMin=[]  SumNumOutMax=[]  DivideOutMin=[]  DivideOutMax=[]  UdiffTsProdOutMin=[]  UdiffTsProdOutMax=[]  NTsProdOutMin=[]  NTsProdOutMax=[]  UintegralTsProdOutMin=[]  UintegralTsProdOutMax=[]  UngainTsProdOutMin=[]  UngainTsProdOutMax=[]  ClampingZeroOutDataTypeStr=Inherit: Inherit via back propagation  ClampingZeroOutMin=[]  ClampingZeroOutMax=[]  FilterDenConstantOutDataTypeStr=Inherit: Inherit via back propagation  FilterDenConstantOutMin=[]  FilterDenConstantOutMax=[]  PCopyOutDataTypeStr=Inherit: Inherit via back propagation  PCopyOutMin=[]  PCopyOutMax=[]  NCopyOutDataTypeStr=Inherit: Inherit via back propagation  NCopyOutMin=[]  NCopyOutMax=[]  IntegratorContinuousStateAttributes=''  IntegratorStateMustResolveToSignalObject=off  IntegratorRTWStateStorageClass=Auto  FilterContinuousStateAttributes=''  FilterStateMustResolveToSignalObject=off  FilterRTWStateStorageClass=Auto  ParallelPVariant=InternalParameters  IdealPVariant=Disabled  IVariant=InternalParameters  DVariant=InternalParameters  IntegratorVariant=Continuous  SatVariant=Enabled  AWVariant=Passthrough  PCopyVariant=Disabled  TRVariant=Disabled  FdbkBlocksVariant=Forward  IdealPFdbkVariant=Disabled  SatFdbkVariant=Disabled  DerivativeFilterVariant=ContFilter  NVariant=InternalParameters  NCopyVariant=Disabled  FilterICVariant=InternalICsFilter  IntegratorICVariant=InternalICs  ExternalResetVariant=Disabled  TRSumVariant=Passthrough  SumFdbkVariant=Disabled  SumVariant=Sum_PID  TsampFilterVariant=InternalTs  TsampNgainVariant=Passthrough  TsampIntegralVariant=Disabled_SignalSpec  ExternalSaturationOutDataTypeStr=Inherit: Same as second input  DerivativeSourceVariant=ErrorSignal
  Constant : Constant  Value=g
  Constant7 : Constant  Value=m
  Derivative1 : Derivative
  Derivative2 : Derivative
  Display1 : Display
  Display2 : Display
  Display3 : Display
  Gain : Gain  Gain=K_z_D2
  Gain1 : Gain  Gain=K_z_P2
  Product4 : Product
  Scope : Scope
  Sum : Sum  Inputs=+++
  Sum1 : Sum  Inputs=|+-
  Sum2 : Sum  Inputs=|-+
  m/cos(y)*(cos(theta)) : MATLAB Function  TreatAsAtomicUnit=on
  target2 : Constant  Value=z_d
  target3 : Constant  Value=z_d
  T : Outport
  wires:
  Product4/1 -> T/1  "T"
  Sum/1 -> Product4/1
  phi/1 -> m/cos(y)*(cos(theta))/2(phi)  "gamma"
  theta/1 -> m/cos(y)*(cos(theta))/3(theta)  "theta"
  Sum2/1 -> Altitude controller/1, Gain1/1
  Derivative2/1 -> Sum1/1
  Constant/1 -> Sum/2
  Derivative1/1 -> Sum1/2
  z/1 -> Derivative1/1, Sum2/1, Display3/1  "z"
  Sum1/1 -> Gain/1
  Constant7/1 -> m/cos(y)*(cos(theta))/1(m)
  m/cos(y)*(cos(theta))/1(c) -> Product4/2
  target2/1 -> Derivative2/1
  Gain/1 -> Display1/1
  target3/1 -> Sum2/2
  Gain1/1 -> Display2/1
  Altitude controller/1 -> Scope/1, Sum/3

== system playground/quad_PID_Simpl2/CONTROLLER/PD regulator gamma1 ==
  phi : Inport
  (phi)' : Inport  Port=2
  Altitude controller1 : slpidlib/PID Controller  Controller=PID  Form=Parallel  TimeDomain=Continuous-time  UseExternalTs=off  SampleTime=-1  IntegratorMethod=Forward Euler  FilterMethod=Forward Euler  ControllerParametersSource=internal  P=K_phi_P22  I=K_phi_I22  UseKiTs=off  D=K_phi_D22  UseExternalDerivativeSource=off  N=100  UseFilter=on  TunerSelectOption=Transfer Function Based (PID Tuner App)  InitialConditionSource=internal  InitialConditionForIntegrator=0  InitialConditionForFilter=0  DifferentiatorICPrevScaledInput=0  ExternalReset=none  TrackingMode=off  Kt=1  LimitOutput=on  SatLimitsSource=internal  UpperSaturationLimit=20  LowerSaturationLimit=-20  LinearizeAsGain=on  AntiWindupMode=none  Kb=1  LimitIntegrator=off  UpperIntegratorSaturationLimit=inf  LowerIntegratorSaturationLimit=-inf  POutMin=[]  POutMax=[]  IOutMin=[]  IOutMax=[]  DOutMin=[]  DOutMax=[]  NOutMin=[]  NOutMax=[]  SumOutMin=[]  SumOutMax=[]  SaturationOutMin=[]  SaturationOutMax=[]  PParamMin=[]  PParamMax=[]  IParamMin=[]  IParamMax=[]  DParamMin=[]  DParamMax=[]  NParamMin=[]  NParamMax=[]  KbParamMin=[]  KbParamMax=[]  KtParamMin=[]  KtParamMax=[]  KbOutMin=[]  KbOutMax=[]  KtOutMin=[]  KtOutMax=[]  IntegratorOutMin=[]  IntegratorOutMax=[]  FilterOutMin=[]  FilterOutMax=[]  SumI1OutMin=[]  SumI1OutMax=[]  SumI2OutMin=[]  SumI2OutMax=[]  SumI3OutMin=[]  SumI3OutMax=[]  SumI4OutMin=[]  SumI4OutMax=[]  SumDOutMin=[]  SumDOutMax=[]  DifferentiatorOutMin=[]  DifferentiatorOutMax=[]  FilterDiffOutCoefMin=[]  FilterDiffOutCoefMax=[]  ReciprocalOutMin=[]  ReciprocalOutMax=[]  SumDenOutMin=[]  SumDenOutMax=[]  SumNumOutMin=[]  SumNumOutMax=[]  DivideOutMin=[]  DivideOutMax=[]  UdiffTsProdOutMin=[]  UdiffTsProdOutMax=[]  NTsProdOutMin=[]  NTsProdOutMax=[]  UintegralTsProdOutMin=[]  UintegralTsProdOutMax=[]  UngainTsProdOutMin=[]  UngainTsProdOutMax=[]  ClampingZeroOutDataTypeStr=Inherit: Inherit via back propagation  ClampingZeroOutMin=[]  ClampingZeroOutMax=[]  FilterDenConstantOutDataTypeStr=Inherit: Inherit via back propagation  FilterDenConstantOutMin=[]  FilterDenConstantOutMax=[]  PCopyOutDataTypeStr=Inherit: Inherit via back propagation  PCopyOutMin=[]  PCopyOutMax=[]  NCopyOutDataTypeStr=Inherit: Inherit via back propagation  NCopyOutMin=[]  NCopyOutMax=[]  IntegratorContinuousStateAttributes=''  IntegratorStateMustResolveToSignalObject=off  IntegratorRTWStateStorageClass=Auto  FilterContinuousStateAttributes=''  FilterStateMustResolveToSignalObject=off  FilterRTWStateStorageClass=Auto  ParallelPVariant=InternalParameters  IdealPVariant=Disabled  IVariant=InternalParameters  DVariant=InternalParameters  IntegratorVariant=Continuous  SatVariant=Enabled  AWVariant=Passthrough  PCopyVariant=Disabled  TRVariant=Disabled  FdbkBlocksVariant=Forward  IdealPFdbkVariant=Disabled  SatFdbkVariant=Disabled  DerivativeFilterVariant=ContFilter  NVariant=InternalParameters  NCopyVariant=Disabled  FilterICVariant=InternalICsFilter  IntegratorICVariant=InternalICs  ExternalResetVariant=Disabled  TRSumVariant=Passthrough  SumFdbkVariant=Disabled  SumVariant=Sum_PID  TsampFilterVariant=InternalTs  TsampNgainVariant=Passthrough  TsampIntegralVariant=Disabled_SignalSpec  ExternalSaturationOutDataTypeStr=Inherit: Same as second input  DerivativeSourceVariant=ErrorSignal
  Constant : Constant  Value=I_x
  Constant2 : Constant  Value=phi_d
  Constant5 : Constant  Value=phi_d
  Current x : Display
  Derivative : Derivative
  Gain : Gain  Gain=K_phi_D2
  Gain1 : Gain  Gain=K_phi_P2
  Manual Switch1 : ManualSwitch
  Manual Switch2 : ManualSwitch
  PID hand : Subsystem
  Product2 : Product
  Scope : Scope
  Scope1 : Scope
  Sum : Sum  Inputs=++|
  Sum1 : Sum  Inputs=|+-
  Sum2 : Sum  Inputs=|+-
  Sum3 : Sum  Inputs=|+-
  Фильтр ПИД1 : TransferFcn  Numerator=[262.14]  Denominator=[K_phi_D22 K_phi_P22 K_phi_I22]
  tau_phi : Outport
  wires:
  Sum/1 -> Current x/1
  Constant/1 -> Product2/2
  (phi)'/1 -> Sum1/2
  Constant2/1 -> Derivative/1
  Derivative/1 -> Scope/1, Sum1/1
  Constant5/1 -> Фильтр ПИД1/1, Sum2/1
  phi/1 -> Sum2/2, Sum3/2
  Sum1/1 -> Gain/1
  Product2/1 -> tau_phi/1  "tau_gamma"
  Gain/1 -> Sum/1
  Sum2/1 -> Manual Switch1/1, Gain1/1
  Gain1/1 -> Sum/2
  Manual Switch1/1 -> PID hand/1(err), Altitude controller1/1
  Фильтр ПИД1/1 -> Sum3/1
  Sum3/1 -> Manual Switch1/2
  Altitude controller1/1 -> Scope1/1, Manual Switch2/2
  Manual Switch2/1 -> Product2/1
  PID hand/1(res) -> Manual Switch2/1

== system playground/quad_PID_Simpl2/CONTROLLER/PD regulator psi ==
  psi : Inport
  (psi)' : Inport  Port=2
  Constant : Constant  Value=I_z
  Constant1 : Constant  Value=K_psi_D2
  Constant2 : Constant  Value=psi_d
  Constant4 : Constant  Value=K_psi_P2
  Constant5 : Constant  Value=psi_d
  Derivative : Derivative
  Manual Switch1 : ManualSwitch
  Manual Switch2 : ManualSwitch  CurrentSetting=0
  Manual Switch3 : ManualSwitch  CurrentSetting=0
  PID hand : Subsystem
  Product : Product
  Product1 : Product
  Product2 : Product
  Scope : Scope
  Sum : Sum  Inputs=++|
  Sum1 : Sum  Inputs=|+-
  Sum2 : Sum  Inputs=|+-
  Sum3 : Sum  Inputs=|+-
  ПИД : slpidlib/PID Controller  Controller=PID  Form=Parallel  TimeDomain=Continuous-time  UseExternalTs=off  SampleTime=-1  IntegratorMethod=Forward Euler  FilterMethod=Forward Euler  ControllerParametersSource=internal  P=K_psi_P22  I=K_psi_I22  UseKiTs=off  D=K_psi_D22  UseExternalDerivativeSource=off  N=100  UseFilter=on  TunerSelectOption=Transfer Function Based (PID Tuner App)  InitialConditionSource=internal  InitialConditionForIntegrator=0  InitialConditionForFilter=0  DifferentiatorICPrevScaledInput=0  ExternalReset=none  TrackingMode=off  Kt=1  LimitOutput=on  SatLimitsSource=internal  UpperSaturationLimit=10  LowerSaturationLimit=-5  LinearizeAsGain=on  AntiWindupMode=none  Kb=1  LimitIntegrator=off  UpperIntegratorSaturationLimit=inf  LowerIntegratorSaturationLimit=-inf  POutMin=[]  POutMax=[]  IOutMin=[]  IOutMax=[]  DOutMin=[]  DOutMax=[]  NOutMin=[]  NOutMax=[]  SumOutMin=[]  SumOutMax=[]  SaturationOutMin=[]  SaturationOutMax=[]  PParamMin=[]  PParamMax=[]  IParamMin=[]  IParamMax=[]  DParamMin=[]  DParamMax=[]  NParamMin=[]  NParamMax=[]  KbParamMin=[]  KbParamMax=[]  KtParamMin=[]  KtParamMax=[]  KbOutMin=[]  KbOutMax=[]  KtOutMin=[]  KtOutMax=[]  IntegratorOutMin=[]  IntegratorOutMax=[]  FilterOutMin=[]  FilterOutMax=[]  SumI1OutMin=[]  SumI1OutMax=[]  SumI2OutMin=[]  SumI2OutMax=[]  SumI3OutMin=[]  SumI3OutMax=[]  SumI4OutMin=[]  SumI4OutMax=[]  SumDOutMin=[]  SumDOutMax=[]  DifferentiatorOutMin=[]  DifferentiatorOutMax=[]  FilterDiffOutCoefMin=[]  FilterDiffOutCoefMax=[]  ReciprocalOutMin=[]  ReciprocalOutMax=[]  SumDenOutMin=[]  SumDenOutMax=[]  SumNumOutMin=[]  SumNumOutMax=[]  DivideOutMin=[]  DivideOutMax=[]  UdiffTsProdOutMin=[]  UdiffTsProdOutMax=[]  NTsProdOutMin=[]  NTsProdOutMax=[]  UintegralTsProdOutMin=[]  UintegralTsProdOutMax=[]  UngainTsProdOutMin=[]  UngainTsProdOutMax=[]  ClampingZeroOutDataTypeStr=Inherit: Inherit via back propagation  ClampingZeroOutMin=[]  ClampingZeroOutMax=[]  FilterDenConstantOutDataTypeStr=Inherit: Inherit via back propagation  FilterDenConstantOutMin=[]  FilterDenConstantOutMax=[]  PCopyOutDataTypeStr=Inherit: Inherit via back propagation  PCopyOutMin=[]  PCopyOutMax=[]  NCopyOutDataTypeStr=Inherit: Inherit via back propagation  NCopyOutMin=[]  NCopyOutMax=[]  IntegratorContinuousStateAttributes=''  IntegratorStateMustResolveToSignalObject=off  IntegratorRTWStateStorageClass=Auto  FilterContinuousStateAttributes=''  FilterStateMustResolveToSignalObject=off  FilterRTWStateStorageClass=Auto  ParallelPVariant=InternalParameters  IdealPVariant=Disabled  IVariant=InternalParameters  DVariant=InternalParameters  IntegratorVariant=Continuous  SatVariant=Enabled  AWVariant=Passthrough  PCopyVariant=Disabled  TRVariant=Disabled  FdbkBlocksVariant=Forward  IdealPFdbkVariant=Disabled  SatFdbkVariant=Disabled  DerivativeFilterVariant=ContFilter  NVariant=InternalParameters  NCopyVariant=Disabled  FilterICVariant=InternalICsFilter  IntegratorICVariant=InternalICs  ExternalResetVariant=Disabled  TRSumVariant=Passthrough  SumFdbkVariant=Disabled  SumVariant=Sum_PID  TsampFilterVariant=InternalTs  TsampNgainVariant=Passthrough  TsampIntegralVariant=Disabled_SignalSpec  ExternalSaturationOutDataTypeStr=Inherit: Same as second input  DerivativeSourceVariant=ErrorSignal
  Фильтр ПИД1 : TransferFcn  Numerator=[max([K_psi_D22 K_psi_P22 K_psi_I22])]  Denominator=[K_psi_D22 K_psi_P22 K_psi_I22]
  tau_psi : Outport
  wires:
  Constant/1 -> Product2/2
  Product2/1 -> tau_psi/1  "tau_psi"
  Sum2/1 -> Manual Switch1/1, Product1/2
  (psi)'/1 -> Sum1/2
  Constant2/1 -> Derivative/1
  Derivative/1 -> Sum1/1
  Constant5/1 -> Фильтр ПИД1/1, Sum2/1
  psi/1 -> Sum2/2, Sum3/2
  Constant4/1 -> Product1/1
  Sum1/1 -> Product/2
  Product1/1 -> Sum/2
  Constant1/1 -> Product/1
  Product/1 -> Sum/1
  Manual Switch1/1 -> PID hand/1(err), ПИД/1
  ПИД/1 -> Manual Switch3/1, Scope/1
  Sum/1 -> Manual Switch2/1
  Manual Switch2/1 -> Product2/1
  Фильтр ПИД1/1 -> Sum3/1
  Sum3/1 -> Manual Switch1/2
  Manual Switch3/1 -> Manual Switch2/2
  PID hand/1(res) -> Manual Switch3/2
